simulink model "XXStIsPosChk"  (R2018b)
settings: Solver=FixedStepDiscrete  StartTime=0.0  StopTime=10.0  FixedStep=0.01  RelTol=1e-3
settings Model: ModifiedHistory=2024.7.4 V3.0.0 557模式流程V1.9  Creator=sn2xws  LastModifiedBy=sn2xws
settings DataIOCC: SaveFormat=StructureWithTime
settings OptimizationCC: DefaultParameterBehavior=Inlined  EnhancedBackFolding=on  PassReuseOutputArgsAs=Individual arguments  ZeroExternalMemoryAtStartup=off  ZeroInternalMemoryAtStartup=off  OptimizeBlockOrder=speed  DifferentSizesBufferReuse=on  OptimizationCustomize=off
settings DebuggingCC: ParameterTunabilityLossMsg=error
settings SFSimCC: MATLABDynamicMemAlloc=off
settings RTWCC: SystemTargetFile=autosar.tlc  GenCodeOnly=on  TemplateMakefile=ert_default_tmf  Description=AUTOSAR  GenerateReport=on  IncludeHyperlinkInReport=on  LaunchReport=on  GenerateTraceInfo=on  GenerateTraceReport=on  GenerateTraceReportSl=on  GenerateTraceReportSf=on  GenerateTraceReportEml=on
settings CodeAppCC: ForceParamTrailComments=on  IgnoreCustomStorageClasses=off  OperatorAnnotations=on  SimulinkDataObjDesc=on  SFDataObjDesc=on  InsertBlockDesc=on
settings STFCustomTargetCC: TargetLangStandard=C99 (ISO)  MultiwordLength=256  ParMdlRefBuildCompliant=on  CompOptLevelCompliant=on  IncludeMdlTerminateFcn=off  CombineOutputUpdateFcns=on  SuppressErrorStatus=on  ERTCustomFileBanners=on  SupportNonFinite=off  SupportComplex=off  SupportContinuousTime=off  SupportNonInlinedSFcns=off  RemoveResetFunc=on  MATLABClassNameForMDSCustomization=Simulink.SoftwareTarget.ERTCustomization  AutosarCompliant=on  UseToolchainInfoCompliant=on  LookupTableObjectStructAxisOrder=2,1,3,4,...  LUTObjectStructOrderEvenSpacing=Size,Table,Breakpoints  SystemTargetFile=autosar.tlc
settings ERTTargetCC: TargetLangStandard=C99 (ISO)  ConcurrentExecutionCompliant=off  IncludeMdlTerminateFcn=off  SuppressErrorStatus=on  SupportNonFinite=off  SupportComplex=off  ModelStepFunctionPrototypeControlCompliant=off  CPPClassGenCompliant=off  AutosarCompliant=on  LookupTableObjectStructAxisOrder=2,1,3,4,...  LUTObjectStructOrderEvenSpacing=Size,Table,Breakpoints  InlinedParameterPlacement=NonHierarchical  ERTCustomFileTemplate=example_file_process.tlc  ERTFilePackagingFormat=Compact

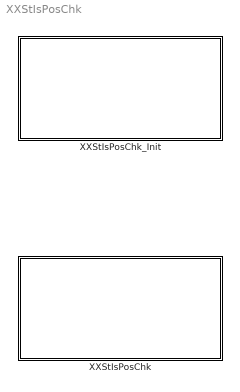
== system XXStIsPosChk ==
  XXStIsPosChk : Subsystem
  XXStIsPosChk_Init : Subsystem

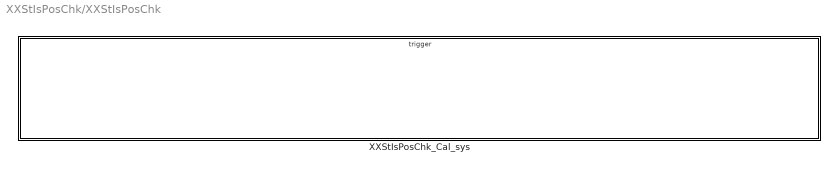
== system XXStIsPosChk/XXStIsPosChk ==
  XXStIsPosChk_Cal_sys : Subsystem

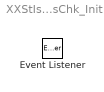
== system XXStIsPosChk/XXStIsPosChk_Init ==
  Event Listener : EventListener  EventName=reset

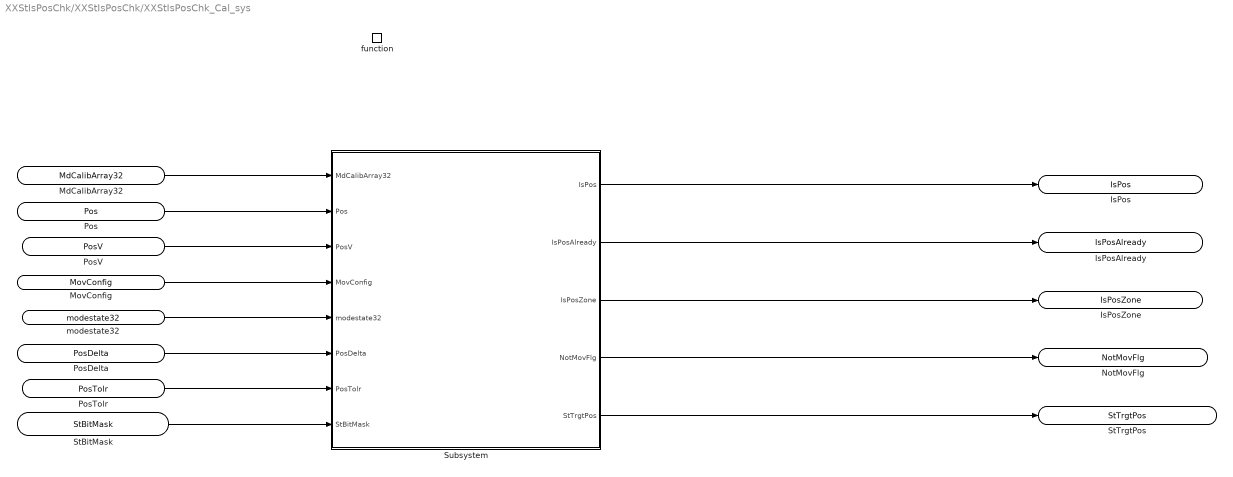
== system XXStIsPosChk/XXStIsPosChk/XXStIsPosChk_Cal_sys ==
  function : TriggerPort  TriggerType=function-call  IsSimulinkFunction=on  FunctionName=XXStIsPosChk_Cal  VariantControl=(inherit)
  Subsystem : Subsystem
  MdCalibArray32 : ArgIn  OutDataTypeStr=uint16  PortDimensions=96  ArgumentName=MdCalibArray32
  Pos : ArgIn  Port=2  OutDataTypeStr=uint16  ArgumentName=Pos
  PosV : ArgIn  Port=3  OutDataTypeStr=boolean  ArgumentName=PosV
  MovConfig : ArgIn  Port=4  OutDataTypeStr=boolean  ArgumentName=MovConfig
  modestate32 : ArgIn  Port=5  OutDataTypeStr=uint32  ArgumentName=modestate32
  PosDelta : ArgIn  Port=6  OutDataTypeStr=uint16  ArgumentName=PosDelta
  PosTolr : ArgIn  Port=7  OutDataTypeStr=uint16  ArgumentName=PosTolr
  StBitMask : ArgIn  Port=8  OutDataTypeStr=uint32  ArgumentName=StBitMask
  IsPos : ArgOut  OutDataTypeStr=uint32  ArgumentName=IsPos
  IsPosAlready : ArgOut  Port=2  OutDataTypeStr=uint32  ArgumentName=IsPosAlready
  IsPosZone : ArgOut  Port=3  OutDataTypeStr=uint32  ArgumentName=IsPosZone
  NotMovFlg : ArgOut  Port=4  OutDataTypeStr=boolean  ArgumentName=NotMovFlg
  StTrgtPos : ArgOut  Port=5  OutDataTypeStr=uint16  ArgumentName=StTrgtPos
  wires:
  MdCalibArray32/1 -> Subsystem/1(MdCalibArray32)
  Pos/1 -> Subsystem/2(Pos)
  PosV/1 -> Subsystem/3(PosV)
  MovConfig/1 -> Subsystem/4(MovConfig)
  modestate32/1 -> Subsystem/5(modestate32)
  PosDelta/1 -> Subsystem/6(PosDelta)
  PosTolr/1 -> Subsystem/7(PosTolr)
  Subsystem/1(IsPos) -> IsPos/1
  Subsystem/2(IsPosAlready) -> IsPosAlready/1
  Subsystem/3(IsPosZone) -> IsPosZone/1
  Subsystem/4(NotMovFlg) -> NotMovFlg/1
  Subsystem/5(StTrgtPos) -> StTrgtPos/1
  StBitMask/1 -> Subsystem/8(StBitMask)

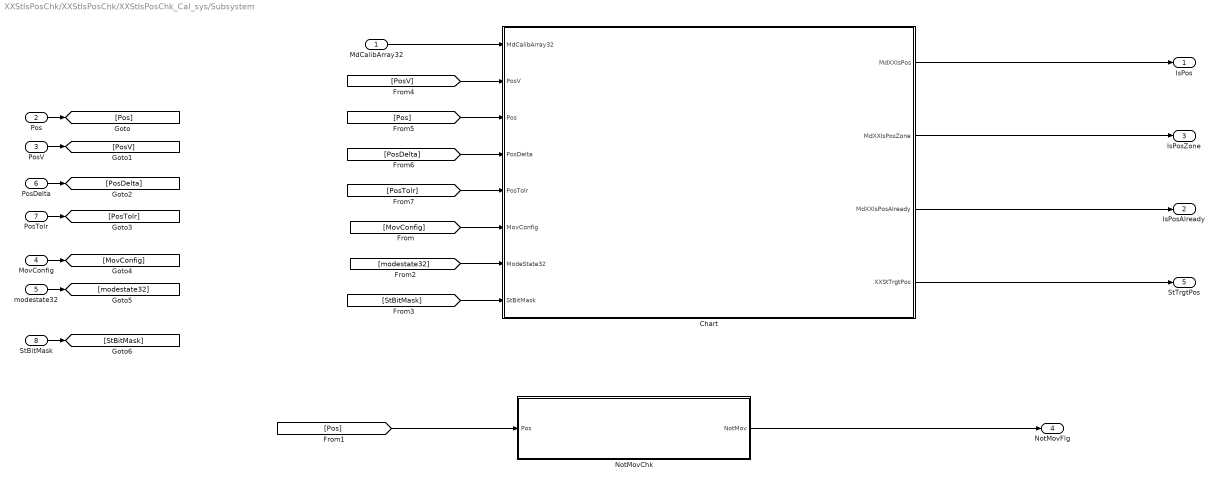
== system XXStIsPosChk/XXStIsPosChk/XXStIsPosChk_Cal_sys/Subsystem ==
  MdCalibArray32 : Inport
  Pos : Inport  Port=2
  PosV : Inport  Port=3
  MovConfig : Inport  Port=4
  modestate32 : Inport  Port=5
  PosDelta : Inport  Port=6
  PosTolr : Inport  Port=7
  StBitMask : Inport  Port=8
  Chart : Stateflow chart  TreatAsAtomicUnit=on
  NotMovChk : Subsystem
  IsPos : Outport
  IsPosAlready : Outport  Port=2
  IsPosZone : Outport  Port=3
  NotMovFlg : Outport  Port=4
  StTrgtPos : Outport  Port=5
  wires:
  MovConfig/1 -> [MovConfig]
  PosV/1 -> [PosV]
  Pos/1 -> [Pos]
  PosDelta/1 -> [PosDelta]
  modestate32/1 -> [modestate32]
  PosTolr/1 -> [PosTolr]
  MdCalibArray32/1 -> Chart/1(MdCalibArray32)
  [PosV] -> Chart/2(PosV)
  [Pos] -> Chart/3(Pos)
  [PosDelta] -> Chart/4(PosDelta)
  [PosTolr] -> Chart/5(PosTolr)
  NotMovChk/1(NotMov) -> NotMovFlg/1
  [Pos] -> NotMovChk/1(Pos)
  [MovConfig] -> Chart/6(MovConfig)
  [modestate32] -> Chart/7(ModeState32)
  Chart/1(MdXXIsPos) -> IsPos/1
  Chart/3(MdXXIsPosAlready) -> IsPosAlready/1
  Chart/4(XXStTrgtPos) -> StTrgtPos/1
  Chart/2(MdXXIsPosZone) -> IsPosZone/1
  StBitMask/1 -> [StBitMask]
  [StBitMask] -> Chart/8(StBitMask)

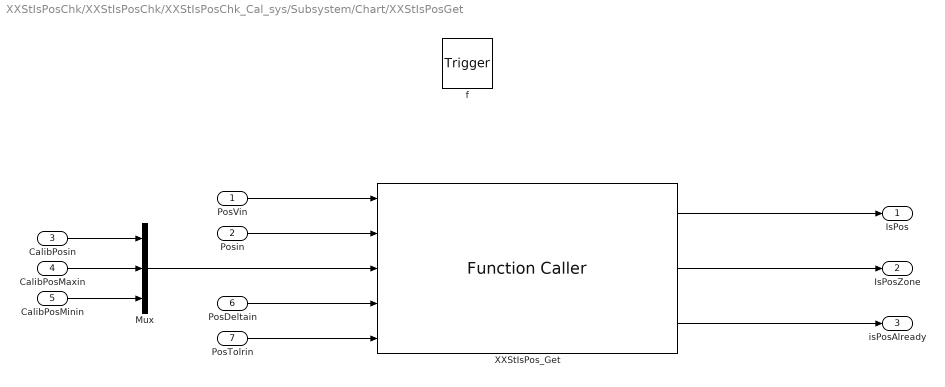
== system XXStIsPosChk/XXStIsPosChk/XXStIsPosChk_Cal_sys/Subsystem/Chart/XXStIsPosGet ==
  PosVin : Inport
  Posin : Inport  Port=2
  CalibPosin : Inport  Port=3
  CalibPosMaxin : Inport  Port=4
  CalibPosMinin : Inport  Port=5
  PosDeltain : Inport  Port=6
  PosTolrin : Inport  Port=7
  f : TriggerPort  TriggerType=function-call  VariantControl=(inherit)
      settings: CopyFcn=Stateflow.SLINSF.SimulinkMan.removeBlockPreDeleteFcn  PreDeleteFcn=Stateflow.SLINSF.SimulinkMan.unsafePredeleteFcn
  Mux : Mux  Inputs=3
  XXStIsPos_Get : FunctionCaller  FunctionPrototype=[IsPos,IsPosZone,IsPosAlready] = XXStIsPos_Get(PosV,Pos,CalibArray,Delta,Tolr)  InputArgumentSpecifications=boolean(true), uint16(1), uint16([1;1;1]), uint16(1), uint16(1)  OutputArgumentSpecifications=boolean(true), boolean(true), boolean(true)
  IsPos : Outport
  IsPosZone : Outport  Port=2
  isPosAlready : Outport  Port=3
  wires:
  PosVin/1 -> XXStIsPos_Get/1
  Posin/1 -> XXStIsPos_Get/2
  PosDeltain/1 -> XXStIsPos_Get/4
  PosTolrin/1 -> XXStIsPos_Get/5
  XXStIsPos_Get/1 -> IsPos/1
  XXStIsPos_Get/2 -> IsPosZone/1
  XXStIsPos_Get/3 -> isPosAlready/1
  Mux/1 -> XXStIsPos_Get/3
  CalibPosin/1 -> Mux/1
  CalibPosMaxin/1 -> Mux/2
  CalibPosMinin/1 -> Mux/3

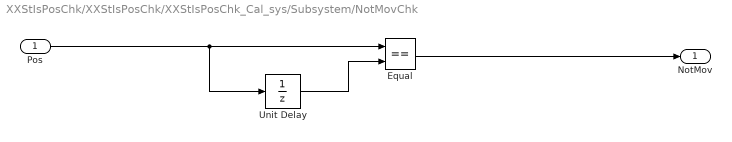
== system XXStIsPosChk/XXStIsPosChk/XXStIsPosChk_Cal_sys/Subsystem/NotMovChk ==
  Pos : Inport
  Equal : RelationalOperator  Operator===  OutDataTypeStr=boolean  RndMeth=Simplest
  Unit Delay : UnitDelay  SampleTime=-1
  NotMov : Outport
  wires:
  Unit Delay/1 -> Equal/2
  Pos/1 -> Unit Delay/1, Equal/1
  Equal/1 -> NotMov/1

== stateflow chart XXStIsPosChk/XXStIsPosChk_Cal_sys/Subsystem/Chart ==
  state [IsPos,IsPosZone,isPosAlready]=XXStIsPosGet(PosVin,Posin,CalibPosin,CalibPosMaxin,CalibPosMinin,PosDeltain,PosTolrin) [function]
  (default) -> (junction 88) : {
      | i=0;
      | MdIsPosArray32 = 0;
      | }
  (junction 88) -> (junction 48) [order 1] : [!MovConfig]
  (junction 88) -> (junction 17) [order 2]
  (junction 48) -> (junction 50) : {
      | MdXXIsPos = 4294967295;
      | MdXXIsPosZone = 4294967295;
      | MdXXIsPosAlready = 4294967295;
      | XXStTrgtPos = 4095;
      | }
  (junction 17) -> (junction 19) [order 1] : [i<32]
  (junction 19) -> (junction 21) : {
      | [TmpIsPos,TmpIsPosZone,TmpIsPosAlready]=XXStIsPosGet(PosV,Pos,MdCalibArray32[i*3],MdCalibArray32[i*3+1],MdCalibArray32[i*3+2],PosDelta,PosTolr);
      | MdIsPosArray32[i*3]= TmpIsPos;
      | MdIsPosArray32[i*3+1] = TmpIsPosZone;
      | MdIsPosArray32[i*3+2] = TmpIsPosAlready;
      | }
  (junction 21) -> (junction 17) : {i=i+1;}
  (junction 17) -> (junction 46) [order 2]
  (junction 46) -> (junction 29) : {
      | i = 0;
      | MdXXIsPos =0x00000000;
      | MdXXIsPosZone = 0x00000000;
      | MdXXIsPosAlready = 0x00000000;
      | }
  (junction 29) -> (junction 41) [order 1] : [i<32]
  (junction 41) -> (junction 43) : {
      | temp_var = uint32(MdIsPosArray32[i*3]);
      | temp_var= temp_var << i;
      | MdXXIsPos = MdXXIsPos |  temp_var;
      | temp_var = uint32(MdIsPosArray32[i*3+1]);
      | temp_var= temp_var << i;
      | MdXXIsPosZone = MdXXIsPos |  temp_var;
      | temp_var = uint32(MdIsPosArray32[i*3+2]);
      | temp_var= temp_var << i;
      | MdXXIsPosAlready = MdXXIsPos |  temp_var;
      | }
  (junction 43) -> (junction 29) : {i=i+1;}
  (junction 29) -> (junction 52) [order 2] : {
      | MdXXIsPos = MdXXIsPos|(~StBitMask);
      | MdXXIsPosZone = MdXXIsPosZone|(~StBitMask);
      | MdXXIsPosAlready = MdXXIsPosAlready|(~StBitMask);
      | }
  (junction 52) -> (junction 56) : {
      | tmpmode32 = ModeState32 & StBitMask;
      | XXStTrgtPos = 4095;
      | }
  (junction 56) -> (junction 62) : {i = 0;}
  (junction 62) -> (junction 69) [order 1] : [i<32]
  (junction 69) -> (junction 71) : {
      | tmpmode32 = ModeState32 & StBitMask
      | tmpmode32 = tmpmode32<< i;
      | }
  (junction 71) -> (junction 62) [order 2] : {i=i+1;}
  (junction 62) -> (junction 66) [order 2]
  (junction 71) -> (junction 74) [order 1] : [(tmpmode32 & 0x00000001)>0]
  (junction 74) -> (junction 76) : {
      | XXStTrgtPos =MdCalibArray32[i*3];
      |  }
  (junction 76) -> (junction 66)
  (junction 50) -> (junction 76)
  (junction 66) -> (junction 82)
  data: PosVin function_input; Posin function_input; CalibPosin function_input; CalibPosMaxin function_input; CalibPosMinin function_input; PosDeltain function_input; PosTolrin function_input; IsPos function_output; IsPosZone function_output; isPosAlready function_output; MdCalibArray32 input; PosV input; Pos input; PosDelta input; PosTolr input; MovConfig input; MdXXIsPos output uint32; MdXXIsPosZone output uint32; MdXXIsPosAlready output uint32; XXStTrgtPos output uint16; ModeState32 input; MdIsPosArray32 local boolean size=96; TmpIsPos local boolean; TmpIsPosZone local boolean; TmpIsPosAlready local boolean; i local uint8; temp_var local uint32; StBitMask input; tmpmode32 local uint32
